simulink model "DTC"  (R2024b)
settings: Solver=ode23tb  StartTime=0.0  StopTime=0.6  RelTol=1e-3
InitFcn:
  | Ts=10e-6;
  | 
  | R=1.2;
  | Ld=5.25e-3;
  | Lq=12e-3;
  | Pn=4;
  | flux=0.175;
libraries: spsDCVoltageSourceLib x1, spsGroundLib x1, spsPermanentMagnetSynchronousMachineLib x1, spsThreePhaseVIMeasurementLib x1, spsUniversalBridgeLib x1, sps_lib x1
settings Model: Creator=23954  LastModifiedBy=23954

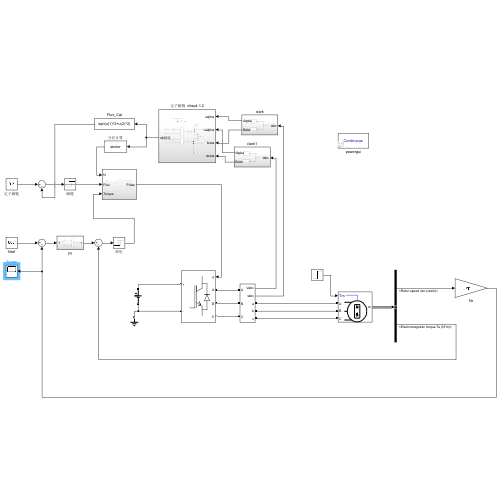
[thumbnail: Simulink's stored preview of the top-level diagram]
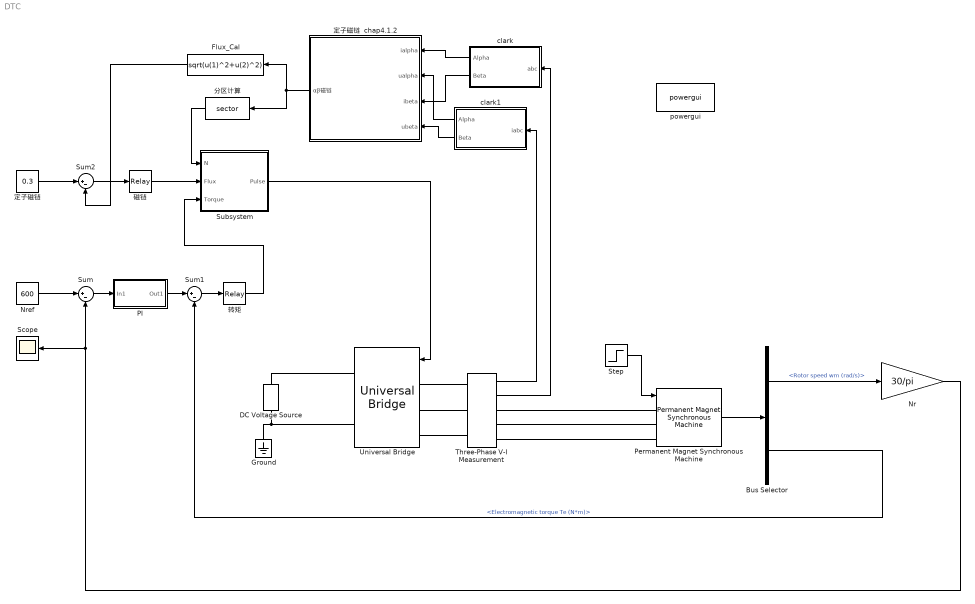
== system DTC ==
  Bus Selector : BusSelector  OutputSignals=Rotor speed wm (rad/s),Electromagnetic torque Te (N*m)
  DC Voltage Source : spsDCVoltageSourceLib/DC Voltage Source  Amplitude=311  Measurements=None
  Flux_Cal : Fcn  Expr=sqrt(u(1)^2+u(2)^2)
  Ground : spsGroundLib/Ground  LConnTagsString=a
  Nr : Gain  Gain=30/pi
  Nref : Constant  Value=600
  PI : Subsystem
  Permanent Magnet Synchronous Machine : spsPermanentMagnetSynchronousMachineLib/Permanent Magnet Synchronous Machine  NbPhases=3  FluxDistribution=Sinusoidal  RotorType=Salient-pole  MechanicalLoad=Torque Tm  PresetModel=No  ShowDetailedParameters=on  MeasurementBus=off  Resistance=1.2  Inductance=8.5e-3  dqInductances=[8.5e-3,8.5e-3]  La=0.000395  MachineConstant=Flux linkage established by magnets (V.s)  Flux=0.175  VoltageCst=126.966  TorqueCst=1.05  Flat=120  Mechanical=[0.0008 0 4]  PolePairs=4  InitialConditions=[0,0, 0,0]  InitialConditions5ph=[0 0 0 0 0 0]  RefAngle=Aligned with phase A axis (original Park)  IterativeDiscreteModel=Trapezoidal non iterative  TsBlock=-1  TsPowergui=0
  Scope : Scope
  Step : Step  Time=0.2  After=1.5  SampleTime=0
  Subsystem : Subsystem
  Sum : Sum  Inputs=|+-
  Sum1 : Sum  Inputs=|+-
  Sum2 : Sum  Inputs=|+-
  Three-Phase V-I Measurement : spsThreePhaseVIMeasurementLib/Three-Phase V-I Measurement  VoltageMeasurement=phase-to-ground  SetLabelV=off  LabelV=Vabc  Vpu=off  VpuLL=off  CurrentMeasurement=yes  SetLabelI=off  LabelI=Iabc  Ipu=off  Pbase=100e6  Vbase=500e3  OutputType=Complex  PhasorSimulation=off  PSBequivalent=0
  Universal Bridge : spsUniversalBridgeLib/Universal Bridge  Arms=3  SnubberResistance=1e5  SnubberCapacitance=inf  Device=IGBT / Diodes  Ron=1e-3  Lon=0  ForwardVoltages="[  0  0  ]"  ForwardVoltage=0  GTOparameters=[ 10e-6 , 20e-6 ]  IGBTparameters=[ 1e-6 , 2e-6 ]  Measurements=None  Measurements_2=None  converterType=Rectifier
  clark : Subsystem
  clark1 : Subsystem
  powergui : sps_lib/powergui  Priority=1  SimulationMode=Continuous  SampleTime=50e-6  frequency=60  Iterations=50  frequencyindice=0  Pbase=100e6  ErrMax=1e-4  UnitsV=kV  UnitsW=MW  buscounter=0  FunctionMessages=off  echomessages=off  EnableUseOfTLC=off  CurrentSourceSwitches=off  DisableSnubberDevices=off  DisableRonSwitches=off  DisableVfSwitches=off  DisplayEquations=off  AutomaticDiscreteSolvers=off  SolverType=Tustin/Backward Euler (TBE)  Interpol=off  ExternalGateDelay=off  methode=off  Ts=100  x0status=blocks  SPID=on  SwTol=0  HookPort=off  NonlinearTolerance=1e-4  nMaxIteration=100  ContinueOnMaxIteration=off  RestoreLinks=warning  ResistiveCurrentMeasurement=off  Frange=[0:2:500]  Ylog=off  Xlog=on  ShowGrid=off  save=off  variable=ZData  structure=0  ZoomFFT=off  StartTime=0.0  cycles=1  DisplayStyle=1  fundamental=60  FreqAxis=off  MaxFrequency=1000  frequencyindicesteady=1  RmsSteady=1  display=off
  分区计算 : S-Function  FunctionName=sector  SFunctionDeploymentMode=off  EnableBusSupport=off
  定子磁链 : Constant  Value=0.3
  定子磁链  chap4.1.2 : Subsystem
  磁链 : Relay  OnSwitchValue=0.002  OffSwitchValue=-0.002
  转矩 : Relay  OnSwitchValue=0.1  OffSwitchValue=-0.1
  wires:
  Step/1 -> Permanent Magnet Synchronous Machine/1
  Permanent Magnet Synchronous Machine/1 -> Bus Selector/1
  Bus Selector/1 -> Nr/1  "<Rotor speed wm (rad/s)>"
  Nref/1 -> Sum/1
  Sum/1 -> PI/1(In1)
  PI/1(Out1) -> Sum1/1
  Bus Selector/2 -> Sum1/2  "<Electromagnetic torque Te (N*m)>"
  Nr/1 -> Scope/1, Sum/2
  Sum1/1 -> 转矩/1
  定子磁链/1 -> Sum2/1
  Sum2/1 -> 磁链/1
  Flux_Cal/1 -> Sum2/2
  转矩/1 -> Subsystem/3(Torque)
  磁链/1 -> Subsystem/2(Flux)
  分区计算/1 -> Subsystem/1(N)
  定子磁链  chap4.1.2/1(αβ磁链) -> 分区计算/1, Flux_Cal/1
  Subsystem/1(Pulse) -> Universal Bridge/1
  Three-Phase V-I Measurement/2 -> clark/1(abc)
  Three-Phase V-I Measurement/1 -> clark1/1(iabc)
  clark/1(Alpha) -> 定子磁链  chap4.1.2/1(ialpha)
  clark/2(Beta) -> 定子磁链  chap4.1.2/3(ibeta)
  clark1/1(Alpha) -> 定子磁链  chap4.1.2/2(ualpha)
  clark1/2(Beta) -> 定子磁链  chap4.1.2/4(ubeta)
  connections:
  DC Voltage Source/RConn1 -- Universal Bridge/RConn1
  DC Voltage Source/LConn1 -- Ground/LConn1 -- Universal Bridge/RConn2
  Three-Phase V-I Measurement/LConn3 -- Universal Bridge/LConn3
  Three-Phase V-I Measurement/LConn2 -- Universal Bridge/LConn2
  Three-Phase V-I Measurement/LConn1 -- Universal Bridge/LConn1
  Permanent Magnet Synchronous Machine/LConn1 -- Three-Phase V-I Measurement/RConn1
  Permanent Magnet Synchronous Machine/LConn2 -- Three-Phase V-I Measurement/RConn2
  Permanent Magnet Synchronous Machine/LConn3 -- Three-Phase V-I Measurement/RConn3

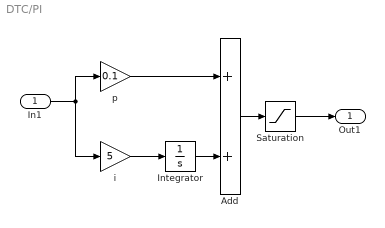
== system DTC/PI ==
  In1 : Inport
  Add : Sum
  Integrator : Integrator
  Saturation : Saturate  UpperLimit=30  LowerLimit=-30
  i : Gain  Gain=5
  p : Gain  Gain=0.1
  Out1 : Outport
  wires:
  i/1 -> Integrator/1
  In1/1 -> p/1, i/1
  p/1 -> Add/1
  Integrator/1 -> Add/2
  Add/1 -> Saturation/1
  Saturation/1 -> Out1/1

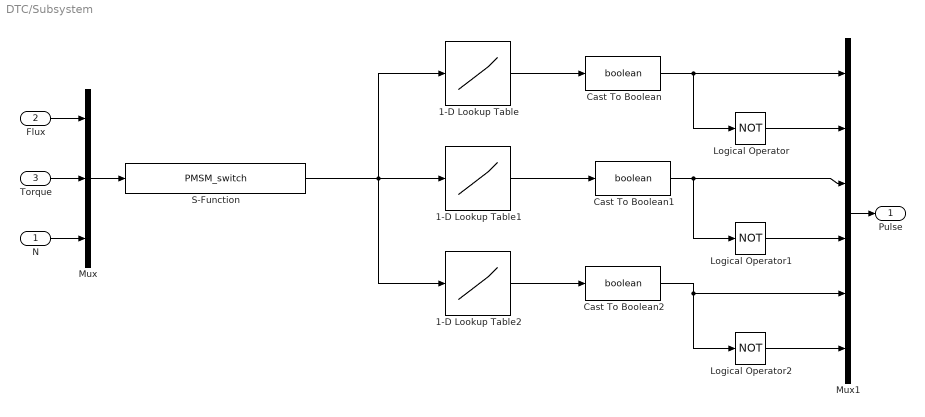
== system DTC/Subsystem ==
  N : Inport
  Flux : Inport  Port=2
  Torque : Inport  Port=3
  1-D Lookup Table : Lookup_n-D  NumberOfTableDimensions=1  BreakpointsForDimension1=[1 2 3 4 5 6]  Table=[1 1 1 0 0 0]  InternalRulePriority=Speed  RndMeth=Simplest
  1-D Lookup Table1 : Lookup_n-D  NumberOfTableDimensions=1  BreakpointsForDimension1=[1 2 3 4 5 6]  Table=[1 0 0 1 1 0]  InternalRulePriority=Speed  RndMeth=Simplest
  1-D Lookup Table2 : Lookup_n-D  NumberOfTableDimensions=1  BreakpointsForDimension1=[1 2 3 4 5 6]  Table=[0 1 0 1 0 1]  InternalRulePriority=Speed  RndMeth=Simplest
  Cast To Boolean : DataTypeConversion  OutDataTypeStr=boolean  SaturateOnIntegerOverflow=off  RndMeth=Floor
  Cast To Boolean1 : DataTypeConversion  OutDataTypeStr=boolean  SaturateOnIntegerOverflow=off  RndMeth=Floor
  Cast To Boolean2 : DataTypeConversion  OutDataTypeStr=boolean  SaturateOnIntegerOverflow=off  RndMeth=Floor
  Logical Operator : Logic  Operator=NOT  AllPortsSameDT=off  OutDataTypeStr=boolean
  Logical Operator1 : Logic  Operator=NOT  AllPortsSameDT=off  OutDataTypeStr=boolean
  Logical Operator2 : Logic  Operator=NOT  AllPortsSameDT=off  OutDataTypeStr=boolean
  Mux : Mux  Inputs=3
  Mux1 : Mux  Inputs=6
  S-Function : S-Function  FunctionName=PMSM_switch  SFunctionDeploymentMode=off  EnableBusSupport=off
  Pulse : Outport
  wires:
  Torque/1 -> Mux/2
  N/1 -> Mux/3
  Flux/1 -> Mux/1
  Mux/1 -> S-Function/1
  S-Function/1 -> 1-D Lookup Table/1, 1-D Lookup Table1/1, 1-D Lookup Table2/1
  1-D Lookup Table/1 -> Cast To Boolean/1
  Cast To Boolean/1 -> Logical Operator/1, Mux1/1
  Logical Operator/1 -> Mux1/2
  Cast To Boolean1/1 -> Logical Operator1/1, Mux1/3
  Logical Operator2/1 -> Mux1/6
  Cast To Boolean2/1 -> Logical Operator2/1, Mux1/5
  Logical Operator1/1 -> Mux1/4
  1-D Lookup Table1/1 -> Cast To Boolean1/1
  1-D Lookup Table2/1 -> Cast To Boolean2/1
  Mux1/1 -> Pulse/1

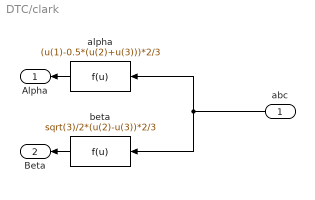
== system DTC/clark ==
  abc : Inport
  alpha : Fcn  Expr=(u(1)-0.5*(u(2)+u(3)))*2/3
  beta : Fcn  Expr=sqrt(3)/2*(u(2)-u(3))*2/3
  Alpha : Outport
  Beta : Outport  Port=2
  wires:
  abc/1 -> alpha/1, beta/1
  alpha/1 -> Alpha/1
  beta/1 -> Beta/1

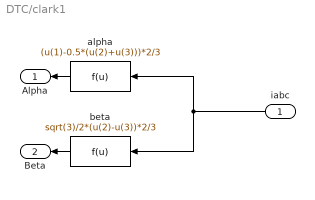
== system DTC/clark1 ==
  iabc : Inport
  alpha : Fcn  Expr=(u(1)-0.5*(u(2)+u(3)))*2/3
  beta : Fcn  Expr=sqrt(3)/2*(u(2)-u(3))*2/3
  Alpha : Outport
  Beta : Outport  Port=2
  wires:
  iabc/1 -> alpha/1, beta/1
  alpha/1 -> Alpha/1
  beta/1 -> Beta/1

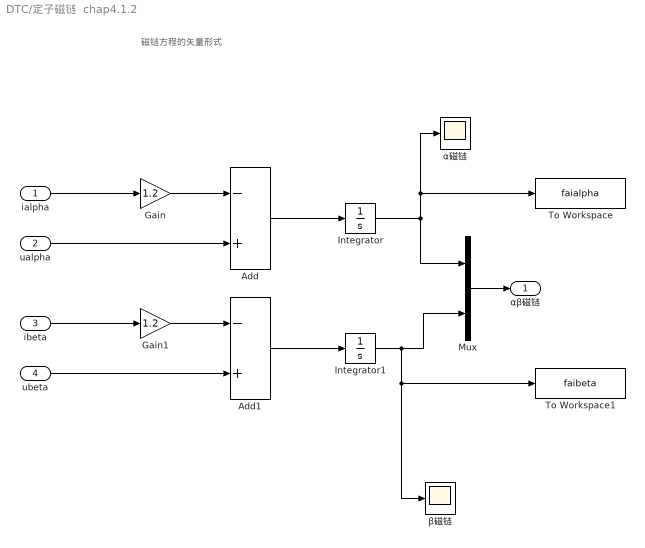
== system DTC/定子磁链  chap4.1.2 ==
  note: 磁链方程的矢量形式
  ialpha : Inport
  ualpha : Inport  Port=2
  ibeta : Inport  Port=3
  ubeta : Inport  Port=4
  Add : Sum  Inputs=-+
  Add1 : Sum  Inputs=-+
  Gain : Gain  Gain=1.2
  Gain1 : Gain  Gain=1.2
  Integrator : Integrator
  Integrator1 : Integrator
  Mux : Mux  Inputs=2
  To Workspace : ToWorkspace  VariableName=faialpha  SampleTime=-1
  To Workspace1 : ToWorkspace  VariableName=faibeta  SampleTime=-1
  α磁链 : Scope
  β磁链 : Scope
  αβ磁链 : Outport
  wires:
  ualpha/1 -> Add/2
  ialpha/1 -> Gain/1
  Gain/1 -> Add/1
  Add/1 -> Integrator/1
  Gain1/1 -> Add1/1
  ibeta/1 -> Gain1/1
  ubeta/1 -> Add1/2
  Add1/1 -> Integrator1/1
  Integrator/1 -> α磁链/1, To Workspace/1, Mux/1
  Integrator1/1 -> β磁链/1, To Workspace1/1, Mux/2
  Mux/1 -> αβ磁链/1
